simulink model "unitdelay"  (Simulink 7.6)
settings: Solver=ode45  StartTime=0.0  StopTime=10.0  RelTol=1e-3
libraries: simulink x1
settings Model: Creator=root  LastModifiedBy=root
settings SolverCC: ZeroCrossAlgorithm=Adaptive

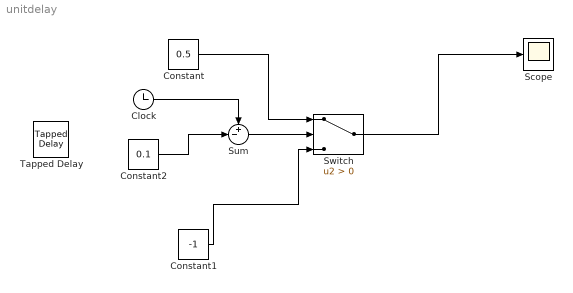
== system unitdelay ==
  Clock : Clock
      settings: Decimation=10
  Constant : Constant  Value=0.5
  Constant1 : Constant  Value=-1
  Constant2 : Constant  Value=0.1
  Scope : Scope
  Sum : Sum  Inputs=+-|
  Switch : Switch  Criteria=u2 > Threshold
  Tapped Delay : simulink/Discrete/Tapped Delay  vinit=0.0  samptime=-1  NumDelays=1  DelayOrder=Oldest  includeCurrent=off
  wires:
  Constant/1 -> Switch/1
  Constant1/1 -> Switch/3
  Sum/1 -> Switch/2
  Clock/1 -> Sum/1
  Constant2/1 -> Sum/2
  Switch/1 -> Scope/1
